simulink model "ManipRoboticoRegolazioneSpazioGiunti"  (R2025b)
settings: Solver=VariableStepAuto  StartTime=0.0  StopTime=10  RelTol=1e-3
values from neighbouring files (symbols this model uses):
  Kd = [15; 15]    [main.m]
  Kp = [20; 20]    [main.m]
settings Model: Creator=arman  LastModifiedBy=arman

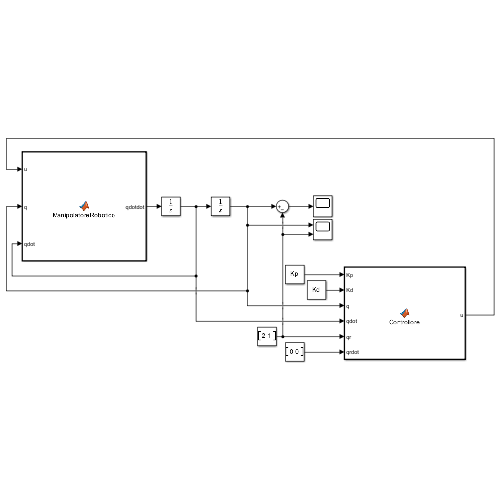
[thumbnail: Simulink's stored preview of the top-level diagram]
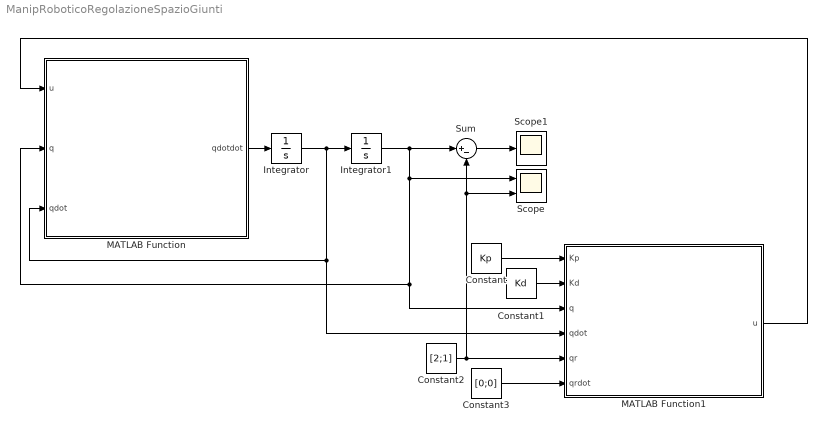
== system ManipRoboticoRegolazioneSpazioGiunti ==
  Constant : Constant  Value=Kp
  Constant1 : Constant  Value=Kd
  Constant2 : Constant  Value=[2;1]
  Constant3 : Constant  Value=[0;0]
  Integrator : Integrator  InitialCondition=[0;0]
  Integrator1 : Integrator  InitialCondition=[0;0]
  MATLAB Function : MATLAB Function  TreatAsAtomicUnit=on
  MATLAB Function1 : MATLAB Function  TreatAsAtomicUnit=on
  Scope : Scope  NumInputPorts=2
      settings: ActiveDisplayYMinimum=-0.28025179159357932  ActiveDisplayYMaximum=2.5222661243422144
  Scope1 : Scope
      settings: ActiveDisplayYMinimum=-0.26556828248960118  ActiveDisplayYMaximum=0.4577536183757544
  Sum : Sum  Inputs=|+-
  wires:
  MATLAB Function/1(qdotdot) -> Integrator/1
  Integrator/1 -> Integrator1/1, MATLAB Function1/4(qdot), MATLAB Function/3(qdot)
  Integrator1/1 -> MATLAB Function1/3(q), MATLAB Function/2(q), Scope/1, Sum/1
  Constant/1 -> MATLAB Function1/1(Kp)
  Constant1/1 -> MATLAB Function1/2(Kd)
  MATLAB Function1/1(u) -> MATLAB Function/1(u)
  Sum/1 -> Scope1/1
  Constant2/1 -> MATLAB Function1/5(qr), Scope/2, Sum/2
  Constant3/1 -> MATLAB Function1/6(qrdot)

== matlab function ManipRoboticoRegolazioneSpazioGiunti/MATLAB Function1 ==
  data: Kp input; Kd input; u output; q input; qdot input; qr input; qrdot input
function u = Controllore(Kp,Kd,q,qdot,qr,qrdot)
e = q - qr;
edot = qdot - qrdot;
[B, C, g, F] = calculateMatrixRobotRR(q,qdot);
u = g - Kd.*edot - Kp.*e;

== matlab function ManipRoboticoRegolazioneSpazioGiunti/MATLAB Function ==
  data: u input; q input; qdotdot output; qdot input
function qdotdot = ManipolatoreRobotico(u,q,qdot)
[B, C, g, F] = calculateMatrixRobotRR(q,qdot);
qdotdot = B \ (u - (C * qdot) - g - F);
